simulink model "SensorProcessingRef"  (R2023b)
settings: Solver=FixedStepDiscrete  StartTime=0.0  StopTime=2  FixedStep=Sample_time  RelTol=1e-3
undefined symbols (not defined in the file): Sample_time, sensor_filter_alpha
Description:
  | Referenced sensor-processing component with a FlightControlBus interface.
settings Model: DataDictionary=FCS_Data.sldd  Creator=Tyler  LastModifiedBy=Tyler
settings CodeAppCC: MaxIdLength=63

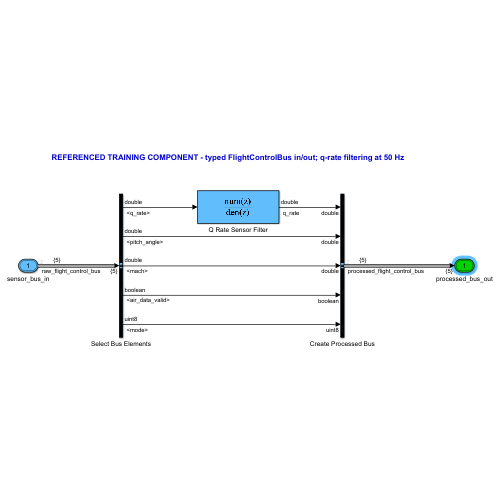
[thumbnail: Simulink's stored preview of the top-level diagram]
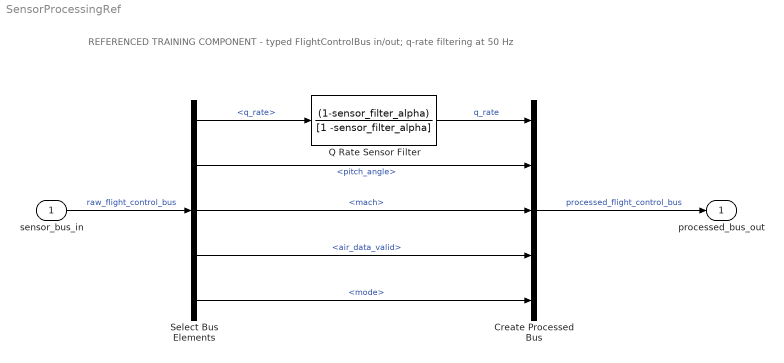
== system SensorProcessingRef ==
  note: REFERENCED TRAINING COMPONENT - typed FlightControlBus in/out; q-rate filtering at 50 Hz
  sensor_bus_in : Inport  OutDataTypeStr=Bus: FlightControlBus  SampleTime=Sample_time
  Create Processed Bus : BusCreator  Inputs=5  OutDataTypeStr=Bus: FlightControlBus
  Q Rate Sensor Filter : DiscreteTransferFcn  Numerator=(1-sensor_filter_alpha)  Denominator=[1 -sensor_filter_alpha]  SampleTime=Sample_time
  Select Bus Elements : BusSelector  OutputSignals=q_rate,pitch_angle,mach,air_data_valid,mode
  processed_bus_out : Outport  OutDataTypeStr=Bus: FlightControlBus
  wires:
  sensor_bus_in/1 -> Select Bus Elements/1  "raw_flight_control_bus"
  Select Bus Elements/1 -> Q Rate Sensor Filter/1  "<q_rate>"
  Q Rate Sensor Filter/1 -> Create Processed Bus/1  "q_rate"
  Select Bus Elements/2 -> Create Processed Bus/2  "<pitch_angle>"
  Select Bus Elements/3 -> Create Processed Bus/3  "<mach>"
  Select Bus Elements/4 -> Create Processed Bus/4  "<air_data_valid>"
  Select Bus Elements/5 -> Create Processed Bus/5  "<mode>"
  Create Processed Bus/1 -> processed_bus_out/1  "processed_flight_control_bus"
